simulink model "satellite_GVE_per_model_formation_sim"  (R2021a)
settings: Solver=VariableStepAuto  StartTime=0  StopTime=10800  FixedStep=1  RelTol=1e-3
values from neighbouring files (symbols this model uses):
  a_ini = (960e3+1019e3)/2+R_e    (= 7367700)    [Satellite_MPC3.m]
  Cd = 2.2    [Satellite_MPC3.m]
  e_ini = 0.0039866    [Satellite_MPC3.m]
  Form_dis = 1e3    (= 1000)    [Satellite_MPC3.m]
  i_ini = 82.9236/180*pi()    [Satellite_MPC3.m]
  J2 = 1082.63e-6    (= 0.00108263)    [Satellite_MPC3.m]
  K = 2    [Satellite_MPC3.m]
  kd = 0    [Satellite_MPC3.m]
  ki = 0    [Satellite_MPC3.m]
  kp = 4e-7    (= 4e-07)    [Satellite_MPC3.m]
  m_s = 27    [Satellite_MPC3.m]
  meu = G*m_e    (= 397865500000000)    [Satellite_MPC3.m]
  Ohm_ini = 272.9481/180*pi()    [Satellite_MPC3.m]
  p_solar = 4.65e-06    [Satellite_MPC3.m]
  R_e = 6378.2e3    (= 6378200)    [Satellite_MPC3.m]
  s = 0.2*0.2    (= 0.04)    [Satellite_MPC3.m]
  theta1_ini = 0    [Satellite_MPC3.m]
  theta2_ini = 1e-7    (= 1e-07)    [Satellite_MPC3.m]
  theta3_ini = 2e-7    (= 2e-07)    [Satellite_MPC3.m]
  theta_ini = 0    [Satellite_MPC3.m]
  u_lim = inf    [Satellite_MPC3.m]
  w_ini = 297.2910/180*pi()    [Satellite_MPC3.m]
libraries: pid_lib x3
(part 1 of 2)
settings Model: OrderedModelArguments=off  Creator=18214  LastModifiedBy=18214

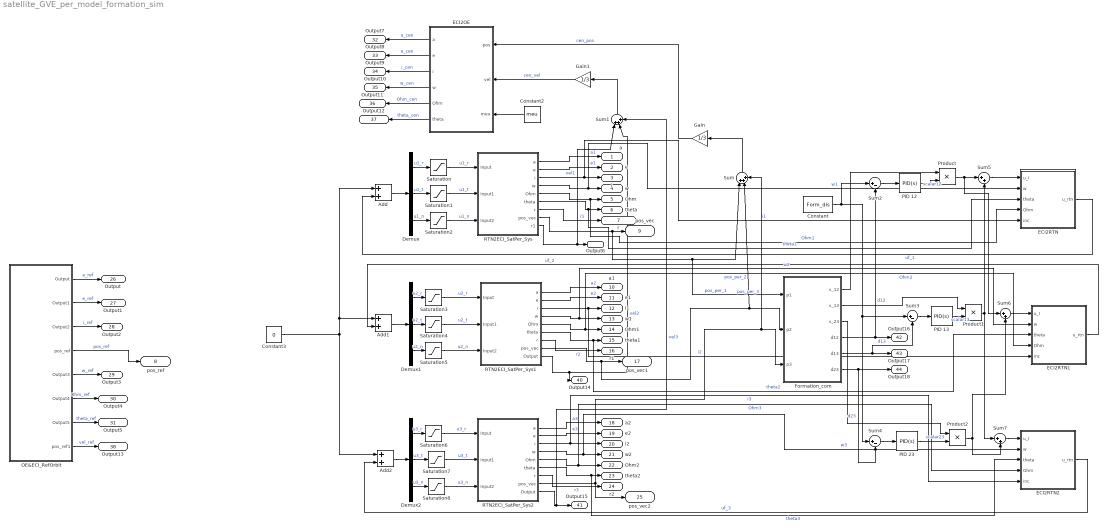
== system satellite_GVE_per_model_formation_sim ==
  Add : Sum
  Add1 : Sum
  Add2 : Sum
  Constant : Constant  Value=Form_dis
  Constant2 : Constant  Value=meu
  Constant3 : Constant  Value=0
  Demux : Demux  Outputs=3
  Demux1 : Demux  Outputs=3
  Demux2 : Demux  Outputs=3
  ECI2OE : MATLAB Function  TreatAsAtomicUnit=on
  ECI2RTN : MATLAB Function  TreatAsAtomicUnit=on
  ECI2RTN1 : MATLAB Function  TreatAsAtomicUnit=on
  ECI2RTN2 : MATLAB Function  TreatAsAtomicUnit=on
  Formation_com : MATLAB Function  TreatAsAtomicUnit=on
  Gain : Gain  Gain=1/3
  Gain1 : Gain  Gain=1/3
  OE&ECI_RefOrbit : Subsystem
  PID 12 : pid_lib/PID Controller  Controller=PID  Form=Parallel  TimeDomain=Continuous-time  UseExternalTs=off  SampleTime=-1  IntegratorMethod=Forward Euler  FilterMethod=Forward Euler  ControllerParametersSource=internal  P=kp  I=ki  D=kd  UseFilter=on  N=100  TunerSelectOption=Transfer Function Based (PID Tuner App)  InitialConditionSource=internal  InitialConditionForIntegrator=0  InitialConditionForFilter=0  DifferentiatorICPrevScaledInput=0  ExternalReset=none  TrackingMode=off  Kt=1  LimitOutput=off  SatLimitsSource=internal  UpperSaturationLimit=inf  LowerSaturationLimit=-inf  LinearizeAsGain=on  AntiWindupMode=none  Kb=1  POutMin=[]  POutMax=[]  IOutMin=[]  IOutMax=[]  DOutMin=[]  DOutMax=[]  NOutMin=[]  NOutMax=[]  SumOutMin=[]  SumOutMax=[]  SaturationOutMin=[]  SaturationOutMax=[]  PParamMin=[]  PParamMax=[]  IParamMin=[]  IParamMax=[]  DParamMin=[]  DParamMax=[]  NParamMin=[]  NParamMax=[]  KbParamMin=[]  KbParamMax=[]  KtParamMin=[]  KtParamMax=[]  KbOutMin=[]  KbOutMax=[]  KtOutMin=[]  KtOutMax=[]  IntegratorOutMin=[]  IntegratorOutMax=[]  FilterOutMin=[]  FilterOutMax=[]  SumI1OutMin=[]  SumI1OutMax=[]  SumI2OutMin=[]  SumI2OutMax=[]  SumI3OutMin=[]  SumI3OutMax=[]  SumI4OutMin=[]  SumI4OutMax=[]  SumDOutMin=[]  SumDOutMax=[]  DifferentiatorOutMin=[]  DifferentiatorOutMax=[]  FilterDiffOutCoefMin=[]  FilterDiffOutCoefMax=[]  ReciprocalOutMin=[]  ReciprocalOutMax=[]  SumDenOutMin=[]  SumDenOutMax=[]  SumNumOutMin=[]  SumNumOutMax=[]  DivideOutMin=[]  DivideOutMax=[]  UdiffTsProdOutMin=[]  UdiffTsProdOutMax=[]  NTsProdOutMin=[]  NTsProdOutMax=[]  UintegralTsProdOutMin=[]  UintegralTsProdOutMax=[]  UngainTsProdOutMin=[]  UngainTsProdOutMax=[]  IntegratorContinuousStateAttributes=''  IntegratorStateMustResolveToSignalObject=off  IntegratorRTWStateStorageClass=Auto  FilterContinuousStateAttributes=''  FilterStateMustResolveToSignalObject=off  FilterRTWStateStorageClass=Auto  ParallelPVariant=InternalParameters  IdealPVariant=Disabled  IVariant=InternalParameters  DVariant=InternalParameters  IntegratorVariant=Continuous  SatVariant=Disabled  AWVariant=Passthrough  PCopyVariant=Disabled  TRVariant=Disabled  FdbkBlocksVariant=Forward  IdealPFdbkVariant=Disabled  SatFdbkVariant=Disabled  DerivativeFilterVariant=ContFilter  NVariant=InternalParameters  NCopyVariant=Disabled  FilterICVariant=InternalICsFilter  IntegratorICVariant=InternalICs  ExternalResetVariant=Disabled  TRSumVariant=Passthrough  SumFdbkVariant=Disabled  SumVariant=Sum_PID  TsampFilterVariant=InternalTs  TsampNgainVariant=Passthrough  TsampIntegralVariant=Passthrough  ExternalSaturationOutDataTypeStr=Inherit: Same as second input
  PID 13 : pid_lib/PID Controller  Controller=PID  Form=Parallel  TimeDomain=Continuous-time  UseExternalTs=off  SampleTime=-1  IntegratorMethod=Forward Euler  FilterMethod=Forward Euler  ControllerParametersSource=internal  P=kp  I=ki  D=kd  UseFilter=on  N=100  TunerSelectOption=Transfer Function Based (PID Tuner App)  InitialConditionSource=internal  InitialConditionForIntegrator=0  InitialConditionForFilter=0  DifferentiatorICPrevScaledInput=0  ExternalReset=none  TrackingMode=off  Kt=1  LimitOutput=off  SatLimitsSource=internal  UpperSaturationLimit=inf  LowerSaturationLimit=-inf  LinearizeAsGain=on  AntiWindupMode=none  Kb=1  POutMin=[]  POutMax=[]  IOutMin=[]  IOutMax=[]  DOutMin=[]  DOutMax=[]  NOutMin=[]  NOutMax=[]  SumOutMin=[]  SumOutMax=[]  SaturationOutMin=[]  SaturationOutMax=[]  PParamMin=[]  PParamMax=[]  IParamMin=[]  IParamMax=[]  DParamMin=[]  DParamMax=[]  NParamMin=[]  NParamMax=[]  KbParamMin=[]  KbParamMax=[]  KtParamMin=[]  KtParamMax=[]  KbOutMin=[]  KbOutMax=[]  KtOutMin=[]  KtOutMax=[]  IntegratorOutMin=[]  IntegratorOutMax=[]  FilterOutMin=[]  FilterOutMax=[]  SumI1OutMin=[]  SumI1OutMax=[]  SumI2OutMin=[]  SumI2OutMax=[]  SumI3OutMin=[]  SumI3OutMax=[]  SumI4OutMin=[]  SumI4OutMax=[]  SumDOutMin=[]  SumDOutMax=[]  DifferentiatorOutMin=[]  DifferentiatorOutMax=[]  FilterDiffOutCoefMin=[]  FilterDiffOutCoefMax=[]  ReciprocalOutMin=[]  ReciprocalOutMax=[]  SumDenOutMin=[]  SumDenOutMax=[]  SumNumOutMin=[]  SumNumOutMax=[]  DivideOutMin=[]  DivideOutMax=[]  UdiffTsProdOutMin=[]  UdiffTsProdOutMax=[]  NTsProdOutMin=[]  NTsProdOutMax=[]  UintegralTsProdOutMin=[]  UintegralTsProdOutMax=[]  UngainTsProdOutMin=[]  UngainTsProdOutMax=[]  IntegratorContinuousStateAttributes=''  IntegratorStateMustResolveToSignalObject=off  IntegratorRTWStateStorageClass=Auto  FilterContinuousStateAttributes=''  FilterStateMustResolveToSignalObject=off  FilterRTWStateStorageClass=Auto  ParallelPVariant=InternalParameters  IdealPVariant=Disabled  IVariant=InternalParameters  DVariant=InternalParameters  IntegratorVariant=Continuous  SatVariant=Disabled  AWVariant=Passthrough  PCopyVariant=Disabled  TRVariant=Disabled  FdbkBlocksVariant=Forward  IdealPFdbkVariant=Disabled  SatFdbkVariant=Disabled  DerivativeFilterVariant=ContFilter  NVariant=InternalParameters  NCopyVariant=Disabled  FilterICVariant=InternalICsFilter  IntegratorICVariant=InternalICs  ExternalResetVariant=Disabled  TRSumVariant=Passthrough  SumFdbkVariant=Disabled  SumVariant=Sum_PID  TsampFilterVariant=InternalTs  TsampNgainVariant=Passthrough  TsampIntegralVariant=Passthrough  ExternalSaturationOutDataTypeStr=Inherit: Same as second input
  PID 23 : pid_lib/PID Controller  Controller=PID  Form=Parallel  TimeDomain=Continuous-time  UseExternalTs=off  SampleTime=-1  IntegratorMethod=Forward Euler  FilterMethod=Forward Euler  ControllerParametersSource=internal  P=kp  I=ki  D=kd  UseFilter=on  N=100  TunerSelectOption=Transfer Function Based (PID Tuner App)  InitialConditionSource=internal  InitialConditionForIntegrator=0  InitialConditionForFilter=0  DifferentiatorICPrevScaledInput=0  ExternalReset=none  TrackingMode=off  Kt=1  LimitOutput=off  SatLimitsSource=internal  UpperSaturationLimit=inf  LowerSaturationLimit=-inf  LinearizeAsGain=on  AntiWindupMode=none  Kb=1  POutMin=[]  POutMax=[]  IOutMin=[]  IOutMax=[]  DOutMin=[]  DOutMax=[]  NOutMin=[]  NOutMax=[]  SumOutMin=[]  SumOutMax=[]  SaturationOutMin=[]  SaturationOutMax=[]  PParamMin=[]  PParamMax=[]  IParamMin=[]  IParamMax=[]  DParamMin=[]  DParamMax=[]  NParamMin=[]  NParamMax=[]  KbParamMin=[]  KbParamMax=[]  KtParamMin=[]  KtParamMax=[]  KbOutMin=[]  KbOutMax=[]  KtOutMin=[]  KtOutMax=[]  IntegratorOutMin=[]  IntegratorOutMax=[]  FilterOutMin=[]  FilterOutMax=[]  SumI1OutMin=[]  SumI1OutMax=[]  SumI2OutMin=[]  SumI2OutMax=[]  SumI3OutMin=[]  SumI3OutMax=[]  SumI4OutMin=[]  SumI4OutMax=[]  SumDOutMin=[]  SumDOutMax=[]  DifferentiatorOutMin=[]  DifferentiatorOutMax=[]  FilterDiffOutCoefMin=[]  FilterDiffOutCoefMax=[]  ReciprocalOutMin=[]  ReciprocalOutMax=[]  SumDenOutMin=[]  SumDenOutMax=[]  SumNumOutMin=[]  SumNumOutMax=[]  DivideOutMin=[]  DivideOutMax=[]  UdiffTsProdOutMin=[]  UdiffTsProdOutMax=[]  NTsProdOutMin=[]  NTsProdOutMax=[]  UintegralTsProdOutMin=[]  UintegralTsProdOutMax=[]  UngainTsProdOutMin=[]  UngainTsProdOutMax=[]  IntegratorContinuousStateAttributes=''  IntegratorStateMustResolveToSignalObject=off  IntegratorRTWStateStorageClass=Auto  FilterContinuousStateAttributes=''  FilterStateMustResolveToSignalObject=off  FilterRTWStateStorageClass=Auto  ParallelPVariant=InternalParameters  IdealPVariant=Disabled  IVariant=InternalParameters  DVariant=InternalParameters  IntegratorVariant=Continuous  SatVariant=Disabled  AWVariant=Passthrough  PCopyVariant=Disabled  TRVariant=Disabled  FdbkBlocksVariant=Forward  IdealPFdbkVariant=Disabled  SatFdbkVariant=Disabled  DerivativeFilterVariant=ContFilter  NVariant=InternalParameters  NCopyVariant=Disabled  FilterICVariant=InternalICsFilter  IntegratorICVariant=InternalICs  ExternalResetVariant=Disabled  TRSumVariant=Passthrough  SumFdbkVariant=Disabled  SumVariant=Sum_PID  TsampFilterVariant=InternalTs  TsampNgainVariant=Passthrough  TsampIntegralVariant=Passthrough  ExternalSaturationOutDataTypeStr=Inherit: Same as second input
  Product : Product
  Product1 : Product
  Product2 : Product
  RTN2ECI_SatPer_Sys : Subsystem
  RTN2ECI_SatPer_Sys1 : Subsystem
  RTN2ECI_SatPer_Sys2 : Subsystem
  Saturation{,1..8} (9 alike) : Saturate  UpperLimit=u_lim  LowerLimit=-u_lim
  Sum : Sum  Inputs=|+++
  Sum1 : Sum  Inputs=|+++
  Sum2 : Sum  Inputs=|+-
  Sum3 : Sum  Inputs=|+-
  Sum4 : Sum  Inputs=|+-
  Sum5 : Sum  Inputs=|++
  Sum6 : Sum  Inputs=|++
  Sum7 : Sum  Inputs=|++
  a : Outport
  e : Outport  Port=2
  i : Outport  Port=3
  w : Outport  Port=4
  Ohm : Outport  Port=5
  theta : Outport  Port=6
  r : Outport  Port=7
  pos_ref : Outport  Port=8
  pos_vec : Outport  Port=9
  a1 : Outport  Port=10
  e1 : Outport  Port=11
  i1 : Outport  Port=12
  w1 : Outport  Port=13
  Ohm1 : Outport  Port=14
  theta1 : Outport  Port=15
  r1 : Outport  Port=16
  pos_vec1 : Outport  Port=17
  a2 : Outport  Port=18
  e2 : Outport  Port=19
  i2 : Outport  Port=20
  w2 : Outport  Port=21
  Ohm2 : Outport  Port=22
  theta2 : Outport  Port=23
  r2 : Outport  Port=24
  pos_vec2 : Outport  Port=25
  Output : Outport  Port=26
  Output1 : Outport  Port=27
  Output2 : Outport  Port=28
  Output3 : Outport  Port=29
  Output4 : Outport  Port=30
  Output5 : Outport  Port=31
  Output7 : Outport  Port=32
  Output8 : Outport  Port=33
  Output9 : Outport  Port=34
  Output10 : Outport  Port=35
  Output11 : Outport  Port=36
  Output12 : Outport  Port=37
  Output13 : Outport  Port=38
  Output6 : Outport  Port=39
  Output14 : Outport  Port=40
  Output15 : Outport  Port=41
  Output16 : Outport  Port=42
  Output17 : Outport  Port=43
  Output18 : Outport  Port=44
  wires:
  Saturation/1 -> RTN2ECI_SatPer_Sys/1(Input)  "u1_r"
  Saturation1/1 -> RTN2ECI_SatPer_Sys/2(Input1)  "u1_t"
  Saturation2/1 -> RTN2ECI_SatPer_Sys/3(Input2)  "u1_n"
  RTN2ECI_SatPer_Sys/1(a) -> a/1  "a1"
  RTN2ECI_SatPer_Sys/2(e) -> e/1  "e1"
  RTN2ECI_SatPer_Sys/3(i) -> ECI2RTN/5(inc), i/1  "i1"
  RTN2ECI_SatPer_Sys/4(w) -> ECI2RTN/2(w), w/1  "w1"
  RTN2ECI_SatPer_Sys/5(Ohm) -> ECI2RTN/4(Ohm), Ohm/1  "Ohm1"
  RTN2ECI_SatPer_Sys/6(theta) -> ECI2RTN/3(theta), theta/1  "theta1"
  RTN2ECI_SatPer_Sys/7(r) -> r/1  "r1"
  RTN2ECI_SatPer_Sys/8(pos_vec) -> Formation_com/1(p1), Sum/1, pos_vec/1  "pos_per_1"
  RTN2ECI_SatPer_Sys1/8(pos_vec) -> Formation_com/2(p2), Sum/2, pos_vec1/1  "pos_per_2"
  RTN2ECI_SatPer_Sys1/7(r) -> r1/1  "r2"
  RTN2ECI_SatPer_Sys1/6(theta) -> ECI2RTN1/3(theta), theta1/1  "theta2"
  RTN2ECI_SatPer_Sys1/5(Ohm) -> ECI2RTN1/4(Ohm), Ohm1/1  "Ohm2"
  RTN2ECI_SatPer_Sys1/4(w) -> ECI2RTN1/2(w), w1/1  "w2"
  RTN2ECI_SatPer_Sys1/3(i) -> ECI2RTN1/5(inc), i1/1  "i2"
  RTN2ECI_SatPer_Sys1/2(e) -> e1/1  "e2"
  RTN2ECI_SatPer_Sys1/1(a) -> a1/1  "a2"
  Saturation5/1 -> RTN2ECI_SatPer_Sys1/3(Input2)  "u2_n"
  Saturation4/1 -> RTN2ECI_SatPer_Sys1/2(Input1)  "u2_t"
  Saturation3/1 -> RTN2ECI_SatPer_Sys1/1(Input)  "u2_r"
  Saturation6/1 -> RTN2ECI_SatPer_Sys2/1(Input)  "u3_r"
  Saturation7/1 -> RTN2ECI_SatPer_Sys2/2(Input1)  "u3_t"
  Saturation8/1 -> RTN2ECI_SatPer_Sys2/3(Input2)  "u3_n"
  RTN2ECI_SatPer_Sys2/1(a) -> a2/1  "a3"
  RTN2ECI_SatPer_Sys2/2(e) -> e2/1  "e3"
  RTN2ECI_SatPer_Sys2/3(i) -> ECI2RTN2/5(inc), i2/1  "i3"
  RTN2ECI_SatPer_Sys2/4(w) -> ECI2RTN2/2(w), w2/1  "w3"
  RTN2ECI_SatPer_Sys2/5(Ohm) -> ECI2RTN2/4(Ohm), Ohm2/1  "Ohm3"
  RTN2ECI_SatPer_Sys2/6(theta) -> ECI2RTN2/3(theta), theta2/1  "theta3"
  RTN2ECI_SatPer_Sys2/7(r) -> r2/1  "r3"
  RTN2ECI_SatPer_Sys2/8(pos_vec) -> pos_vec2/1, Formation_com/3(p3), Sum/3  "pos_per_3"
  OE&ECI_RefOrbit/1(Output) -> Output/1  "a_ref"
  OE&ECI_RefOrbit/2(Output1) -> Output1/1  "e_ref"
  OE&ECI_RefOrbit/3(Output2) -> Output2/1  "i_ref"
  OE&ECI_RefOrbit/4(pos_ref) -> pos_ref/1  "pos_ref"
  OE&ECI_RefOrbit/5(Output3) -> Output3/1  "w_ref"
  OE&ECI_RefOrbit/6(Output4) -> Output4/1  "Ohm_ref"
  OE&ECI_RefOrbit/7(Output5) -> Output5/1  "theta_ref"
  Constant/1 -> Sum3/1, Sum4/1, Sum2/1
  Sum/1 -> Gain/1
  Add/1 -> Demux/1
  Add1/1 -> Demux1/1
  Add2/1 -> Demux2/1
  Constant3/1 -> Add2/1, Add/1, Add1/1
  Gain/1 -> ECI2OE/1(pos)  "cen_pos"
  Constant2/1 -> ECI2OE/3(meu)
  ECI2OE/1(a) -> Output7/1  "a_cen"
  ECI2OE/2(e) -> Output8/1  "e_cen"
  ECI2OE/3(i) -> Output9/1  "i_cen"
  ECI2OE/4(w) -> Output10/1  "w_cen"
  ECI2OE/5(Ohm) -> Output11/1  "Ohm_cen"
  ECI2OE/6(theta) -> Output12/1  "theta_cen"
  OE&ECI_RefOrbit/8(pos_ref1) -> Output13/1  "vel_ref"
  RTN2ECI_SatPer_Sys/9(r1) -> Sum1/1, Output6/1  "vel1"
  RTN2ECI_SatPer_Sys1/9(Output) -> Sum1/2, Output14/1  "vel2"
  RTN2ECI_SatPer_Sys2/9(Output) -> Sum1/3, Output15/1  "vel3"
  Gain1/1 -> ECI2OE/2(vel)  "cen_vel"
  Sum1/1 -> Gain1/1
  ECI2RTN/1(u_rtn) -> Add/2  "uf_1"
  Sum3/1 -> PID 13/1
  ECI2RTN1/1(u_rtn) -> Add1/2  "uf_2"
  Demux/1 -> Saturation/1  "u1_r"
  Demux/2 -> Saturation1/1  "u1_t"
  Demux/3 -> Saturation2/1  "u1_n"
  Demux1/1 -> Saturation3/1  "u2_r"
  Demux1/2 -> Saturation4/1  "u2_t"
  Demux1/3 -> Saturation5/1  "u2_n"
  Demux2/1 -> Saturation6/1  "u3_r"
  Demux2/2 -> Saturation7/1  "u3_t"
  Demux2/3 -> Saturation8/1  "u3_n"
  Sum4/1 -> PID 23/1
  ECI2RTN2/1(u_rtn) -> Add2/2  "uf_3"
  Formation_com/4(d12) -> Output16/1, Sum2/2  "d12"
  Formation_com/5(d13) -> Sum3/2, Output17/1  "d13"
  Formation_com/6(d23) -> Sum4/2, Output18/1  "d23"
  Sum5/1 -> ECI2RTN/1(u_I)
  Product1/1 -> Sum5/2, Sum7/1
  Sum7/1 -> ECI2RTN2/1(u_I)
  Sum2/1 -> PID 12/1
  PID 12/1 -> Product/2  "scalar12"
  Formation_com/1(v_12) -> Product/1
  PID 13/1 -> Product1/2  "scalar13"
  Formation_com/2(v_13) -> Product1/1
  PID 23/1 -> Product2/2  "scalar23"
  Formation_com/3(v_23) -> Product2/1
  Product/1 -> Sum6/1, Sum5/1
  Sum6/1 -> ECI2RTN1/1(u_I)
  Product2/1 -> Sum6/2, Sum7/2

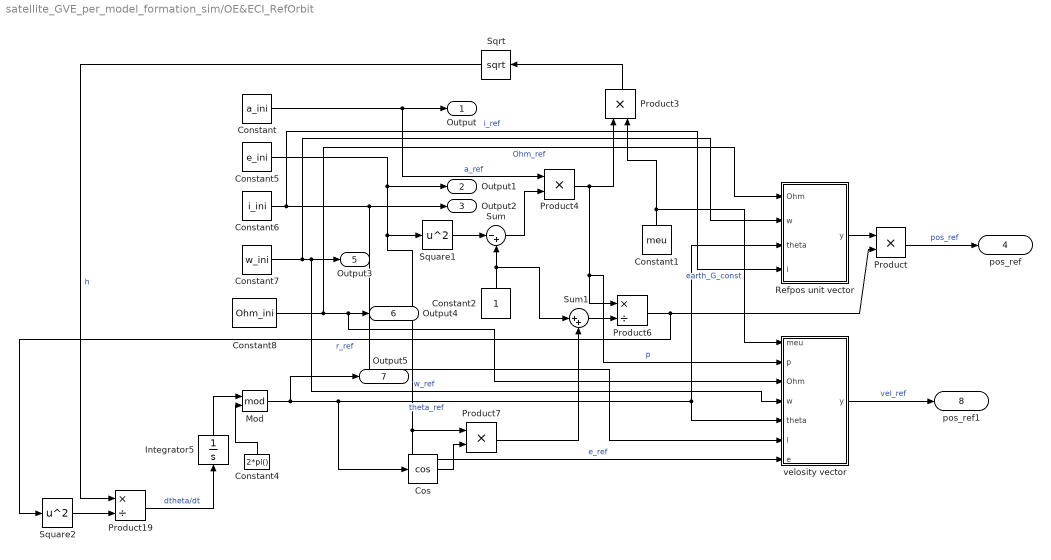
== system satellite_GVE_per_model_formation_sim/OE&ECI_RefOrbit ==
  Constant : Constant  Value=a_ini
  Constant1 : Constant  Value=meu
  Constant2 : Constant
  Constant4 : Constant  Value=2*pi()
  Constant5 : Constant  Value=e_ini
  Constant6 : Constant  Value=i_ini
  Constant7 : Constant  Value=w_ini
  Constant8 : Constant  Value=Ohm_ini
  Cos : Trigonometry  Operator=cos
  Integrator5 : Integrator  InitialCondition=theta_ini
  Mod : Math  Operator=mod  SaturateOnIntegerOverflow=on
  Product{,3..4,7} (4 alike) : Product
  Product19 : Product  Inputs=*/
  Product6 : Product  Inputs=*/
  Refpos unit vector : MATLAB Function  TreatAsAtomicUnit=on
  Sqrt : Sqrt  SaturateOnIntegerOverflow=on
  Square1 : Math  Operator=square  SaturateOnIntegerOverflow=on
  Square2 : Math  Operator=square  SaturateOnIntegerOverflow=on
  Sum : Sum  Inputs=|-+
  Sum1 : Sum  Inputs=|++
  velosity vector : MATLAB Function  TreatAsAtomicUnit=on
  Output : Outport
  Output1 : Outport  Port=2
  Output2 : Outport  Port=3
  pos_ref : Outport  Port=4
  Output3 : Outport  Port=5
  Output4 : Outport  Port=6
  Output5 : Outport  Port=7
  pos_ref1 : Outport  Port=8
  wires:
  Constant/1 -> Output/1, Product4/1  "a_ref"
  Constant6/1 -> velosity vector/6(i), Output2/1, Refpos unit vector/4(i)  "i_ref"
  Constant7/1 -> velosity vector/4(w), Output3/1, Refpos unit vector/2(w)  "w_ref"
  Product6/1 -> Product/2, Square2/1  "r_ref"
  Constant8/1 -> velosity vector/3(Ohm), Output4/1, Refpos unit vector/1(Ohm)  "Ohm_ref"
  Constant2/1 -> Sum/2, Sum1/1
  Refpos unit vector/1(y) -> Product/1
  Product/1 -> pos_ref/1  "pos_ref"
  Product7/1 -> Sum1/2
  Product4/1 -> velosity vector/2(p), Product6/1, Product3/1  "p"
  Cos/1 -> Product7/2
  Mod/1 -> Output5/1, velosity vector/5(theta), Refpos unit vector/3(theta), Cos/1  "theta_ref"
  Integrator5/1 -> Mod/1
  Square1/1 -> Sum/1
  Sqrt/1 -> Product19/1  "h"
  Constant5/1 -> Output1/1, Product7/1, velosity vector/7(e), Square1/1  "e_ref"
  Sum/1 -> Product4/2
  Constant4/1 -> Mod/2
  Product3/1 -> Sqrt/1
  Product19/1 -> Integrator5/1  "dtheta/dt"
  Constant1/1 -> Product3/2, velosity vector/1(meu)  "earth_G_const"
  Square2/1 -> Product19/2
  Sum1/1 -> Product6/2
  velosity vector/1(y) -> pos_ref1/1  "vel_ref"

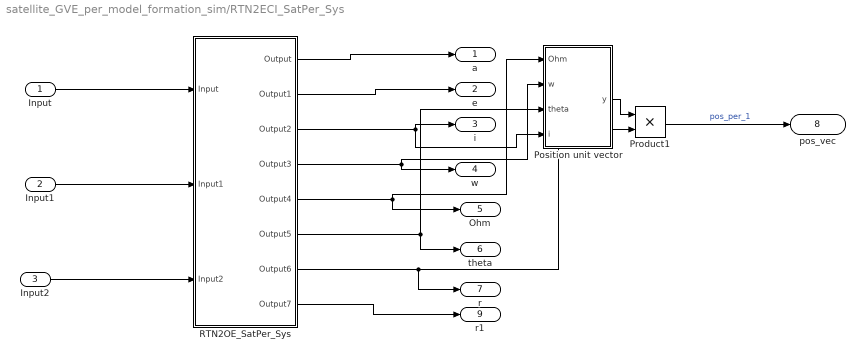
== system satellite_GVE_per_model_formation_sim/RTN2ECI_SatPer_Sys ==
  Input : Inport
  Input1 : Inport  Port=2
  Input2 : Inport  Port=3
  Position unit vector : MATLAB Function  TreatAsAtomicUnit=on
  Product1 : Product
  RTN2OE_SatPer_Sys : Subsystem
  a : Outport
  e : Outport  Port=2
  i : Outport  Port=3
  w : Outport  Port=4
  Ohm : Outport  Port=5
  theta : Outport  Port=6
  r : Outport  Port=7
  pos_vec : Outport  Port=8
  r1 : Outport  Port=9
  wires:
  Position unit vector/1(y) -> Product1/1
  RTN2OE_SatPer_Sys/6(Output5) -> theta/1, Position unit vector/3(theta)
  RTN2OE_SatPer_Sys/4(Output3) -> w/1, Position unit vector/2(w)
  Product1/1 -> pos_vec/1  "pos_per_1"
  RTN2OE_SatPer_Sys/2(Output1) -> e/1
  RTN2OE_SatPer_Sys/5(Output4) -> Ohm/1, Position unit vector/1(Ohm)
  RTN2OE_SatPer_Sys/7(Output6) -> r/1, Product1/2
  RTN2OE_SatPer_Sys/1(Output) -> a/1
  RTN2OE_SatPer_Sys/3(Output2) -> Position unit vector/4(i), i/1
  Input/1 -> RTN2OE_SatPer_Sys/1(Input)
  Input1/1 -> RTN2OE_SatPer_Sys/2(Input1)
  Input2/1 -> RTN2OE_SatPer_Sys/3(Input2)
  RTN2OE_SatPer_Sys/8(Output7) -> r1/1

== system satellite_GVE_per_model_formation_sim/RTN2ECI_SatPer_Sys1 ==
  Input : Inport
  Input1 : Inport  Port=2
  Input2 : Inport  Port=3
  Position unit vector : MATLAB Function  TreatAsAtomicUnit=on
  Product1 : Product
  RTN2OE_SatPer_Sys : Subsystem
  a : Outport
  e : Outport  Port=2
  i : Outport  Port=3
  w : Outport  Port=4
  Ohm : Outport  Port=5
  theta : Outport  Port=6
  r : Outport  Port=7
  pos_vec : Outport  Port=8
  Output : Outport  Port=9
  wires:
  RTN2OE_SatPer_Sys/3(Output2) -> Position unit vector/4(i), i/1
  RTN2OE_SatPer_Sys/1(Output) -> a/1
  RTN2OE_SatPer_Sys/7(Output6) -> r/1, Product1/2
  RTN2OE_SatPer_Sys/5(Output4) -> Position unit vector/1(Ohm), Ohm/1
  RTN2OE_SatPer_Sys/2(Output1) -> e/1
  Product1/1 -> pos_vec/1  "pos_per_2"
  RTN2OE_SatPer_Sys/4(Output3) -> Position unit vector/2(w), w/1
  RTN2OE_SatPer_Sys/6(Output5) -> theta/1, Position unit vector/3(theta)
  Position unit vector/1(y) -> Product1/1
  Input/1 -> RTN2OE_SatPer_Sys/1(Input)
  Input1/1 -> RTN2OE_SatPer_Sys/2(Input1)
  Input2/1 -> RTN2OE_SatPer_Sys/3(Input2)
  RTN2OE_SatPer_Sys/8(Output7) -> Output/1

== system satellite_GVE_per_model_formation_sim/RTN2ECI_SatPer_Sys2 ==
  Input : Inport
  Input1 : Inport  Port=2
  Input2 : Inport  Port=3
  Position unit vector : MATLAB Function  TreatAsAtomicUnit=on
  Product1 : Product
  RTN2OE_SatPer_Sys : Subsystem
  a : Outport
  e : Outport  Port=2
  i : Outport  Port=3
  w : Outport  Port=4
  Ohm : Outport  Port=5
  theta : Outport  Port=6
  r : Outport  Port=7
  pos_vec : Outport  Port=8
  Output : Outport  Port=9
  wires:
  Position unit vector/1(y) -> Product1/1
  RTN2OE_SatPer_Sys/6(Output5) -> theta/1, Position unit vector/3(theta)
  RTN2OE_SatPer_Sys/4(Output3) -> w/1, Position unit vector/2(w)
  Product1/1 -> pos_vec/1  "pos_per_3"
  RTN2OE_SatPer_Sys/2(Output1) -> e/1
  RTN2OE_SatPer_Sys/5(Output4) -> Ohm/1, Position unit vector/1(Ohm)
  RTN2OE_SatPer_Sys/7(Output6) -> r/1, Product1/2
  RTN2OE_SatPer_Sys/1(Output) -> a/1
  RTN2OE_SatPer_Sys/3(Output2) -> i/1, Position unit vector/4(i)
  Input/1 -> RTN2OE_SatPer_Sys/1(Input)
  Input1/1 -> RTN2OE_SatPer_Sys/2(Input1)
  Input2/1 -> RTN2OE_SatPer_Sys/3(Input2)
  RTN2OE_SatPer_Sys/8(Output7) -> Output/1

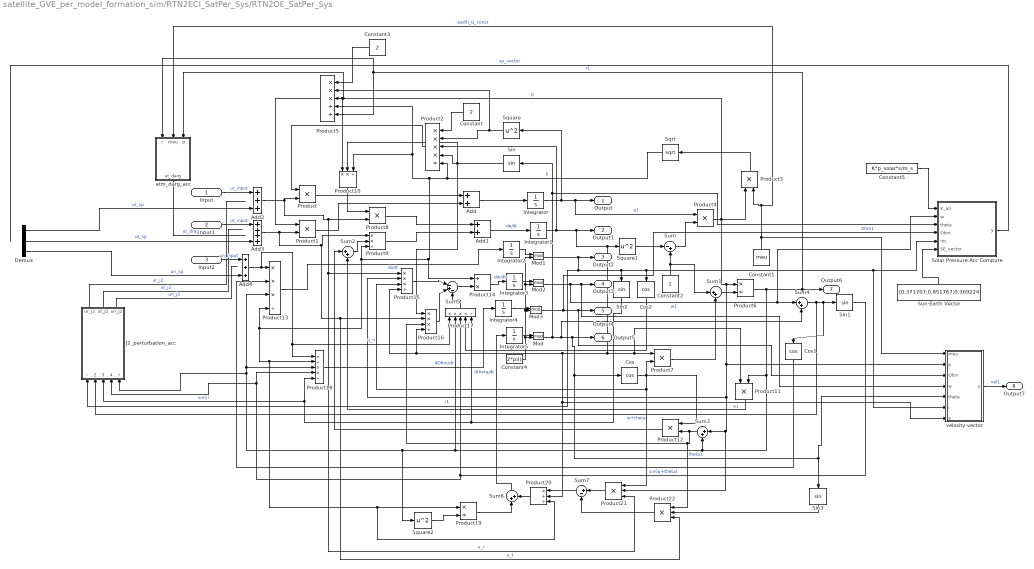
== system satellite_GVE_per_model_formation_sim/RTN2ECI_SatPer_Sys/RTN2OE_SatPer_Sys ==
  Input : Inport
  Input1 : Inport  Port=2
  Input2 : Inport  Port=3
  Add : Sum
  Add1 : Sum
  Add2 : Sum  Inputs=+++
  Add3 : Sum  Inputs=++++
  Add4 : Sum  Inputs=+++
  Constant : Constant  Value=2
  Constant1 : Constant  Value=meu
  Constant2 : Constant
  Constant3 : Constant  Value=2
  Constant4 : Constant  Value=2*pi()
  Constant5 : Constant  Value=K*p_solar*s/m_s
  Cos : Trigonometry  Operator=cos
  Cos1 : Trigonometry  Operator=cos
  Cos2 : Trigonometry  Operator=cos
  Demux : Demux  Outputs=3
  Integrator : Integrator  InitialCondition=a_ini  LimitOutput=on  LowerSaturationLimit=R_e
  Integrator1 : Integrator  InitialCondition=e_ini  LimitOutput=on  UpperSaturationLimit=1  LowerSaturationLimit=0
  Integrator2 : Integrator  InitialCondition=i_ini  UpperSaturationLimit=312.5963  LowerSaturationLimit=-312.5963
  Integrator3 : Integrator  InitialCondition=w_ini  UpperSaturationLimit=312.5963  LowerSaturationLimit=-312.5963
  Integrator4 : Integrator  InitialCondition=Ohm_ini  UpperSaturationLimit=312.5963  LowerSaturationLimit=-312.5963
  Integrator5 : Integrator  InitialCondition=theta1_ini  UpperSaturationLimit=312.5963  LowerSaturationLimit=-312.5963
  J2_perturbation_acc : Subsystem
  Mod{,1..3} (4 alike) : Math  Operator=mod  SaturateOnIntegerOverflow=on
  Product{,1,3..4,7..8,11..12} (8 alike) : Product
  Product10 : Product  Inputs=**/
  Product13 : Product  Inputs=***/
  Product14 : Product  Inputs=/*
  Product15 : Product  Inputs=***/
  Product16 : Product  Inputs=***/
  Product17 : Product  Inputs=****/
  Product18 : Product  Inputs=*/**/
  Product19 : Product  Inputs=*/
  Product2 : Product  Inputs=****/
  Product20 : Product  Inputs=*//
  Product21 : Product  Inputs=***
  Product22 : Product  Inputs=***
  Product5 : Product  Inputs=***//
  Product6 : Product  Inputs=*/
  Product9 : Product  Inputs=**/
  Sin{,1..3} (4 alike) : Trigonometry
  Solar Pressure Acc Compute : MATLAB Function  TreatAsAtomicUnit=on
  Sqrt : Sqrt  SaturateOnIntegerOverflow=on
  Square : Math  Operator=square  SaturateOnIntegerOverflow=on
  Square1 : Math  Operator=square  SaturateOnIntegerOverflow=on
  Square2 : Math  Operator=square  SaturateOnIntegerOverflow=on
  Sum : Sum  Inputs=|-+
  Sum{1..4,6} (5 alike) : Sum  Inputs=|++
  Sum5 : Sum  Inputs=|-+-
  Sum7 : Sum  Inputs=|+-
  Sun-Earth Vector : Constant  Value=[0.371707;0.851767;0.369224]
  atm_darg_acc : Subsystem
  velosity vector : MATLAB Function  TreatAsAtomicUnit=on
  Output : Outport
  Output1 : Outport  Port=2
  Output2 : Outport  Port=3
  Output3 : Outport  Port=4
  Output4 : Outport  Port=5
  Output5 : Outport  Port=6
  Output6 : Outport  Port=7
  Output7 : Outport  Port=8
  wires:
  Integrator/1 -> Output/1, Product4/1, Square/1  "a1"
  Square2/1 -> Product19/2
  Product2/1 -> Product/1
  Mod/1 -> Sin/1, Solar Pressure Acc Compute/3(theta), Output5/1, Sin3/1, velosity vector/5(theta), Cos/1, Sum4/2  "theta1"
  Sin1/1 -> Product18/4, J2_perturbation_acc/4(sin(w+theta)), Product17/3  "sin(w+theta)"
  Product21/1 -> Sum7/1
  Sum5/1 -> Product14/2
  Cos/1 -> Product21/1, Product15/3, Product12/1, Product7/2
  Product4/1 -> Product15/2, Product21/2, Sum3/1, velosity vector/2(p), Product6/1, atm_darg_acc/3(p), Product10/1, Product5/3, Product3/1  "p"
  Cos2/1 -> Product17/4
  Sin/1 -> Product16/1, Product10/2, Product2/4
  Sqrt/1 -> Product10/3, Product5/4, Product14/1, Product13/4, Product20/3, Product19/1, Product18/2, Product9/3, Product2/5  "h"
  Product12/1 -> Sum2/1
  Sum/1 -> Product4/2
  Sum3/1 -> Product22/1, Product16/3, Product12/2
  Sum7/1 -> Product20/1
  Product1/1 -> Add/2
  Product22/1 -> Sum7/2
  Add2/1 -> Product/2, Product21/3, Product15/1, Product8/2  "u_r"
  Product7/1 -> Sum1/2
  Product5/1 -> Product1/1
  Sin3/1 -> Product22/2
  Product15/1 -> Sum5/1
  Integrator1/1 -> Product2/3, Output1/1, Square1/1, Product7/1, Product11/1, Product20/2, velosity vector/7(e), Product16/4, Product15/4  "e1"
  Sum1/1 -> Product6/2
  Cos1/1 -> Product13/2
  Product19/1 -> Sum6/1
  Product8/1 -> Add1/1
  Product6/1 -> atm_darg_acc/1(r), Product5/5, Output6/1, Square2/1, J2_perturbation_acc/5(r), Product13/3, Product18/3, Product17/2, Sum3/2, Product11/2  "r1"
  Constant2/1 -> Sum/2, Sum1/1
  Square/1 -> Product5/2, Product2/2
  Product11/1 -> Sum2/2
  Product/1 -> Add/1
  Mod1/1 -> Output2/1, velosity vector/6(i), Solar Pressure Acc Compute/5(inc), Cos2/1, Sin2/1, J2_perturbation_acc/1(i)  "i1"
  Sin2/1 -> Product18/5, J2_perturbation_acc/3(sin(i)), Product17/5  "sin(i)"
  Product17/1 -> Sum5/3
  Product16/1 -> Sum5/2
  Sum6/1 -> Integrator5/1  "dtheta/dt"
  Product10/1 -> Product8/1
  Product9/1 -> Add1/2
  Sum4/1 -> Sin1/1, Cos1/1, J2_perturbation_acc/2(w+theta)  "w+theta"
  Product20/1 -> Sum6/2
  Mod2/1 -> Solar Pressure Acc Compute/2(w), Sum4/1, velosity vector/4(w), Output3/1  "w1"
  Add3/1 -> Product22/3, Product16/2, Product9/1, Product1/2  "u_t"
  Constant/1 -> Product2/1
  Sum2/1 -> Product9/2
  Product14/1 -> Integrator3/1  "dw/dt"
  Square1/1 -> Sum/1
  Add4/1 -> Product18/1, Product17/1, Product13/1  "u_n"
  Product13/1 -> Integrator2/1  "di/dt"
  Constant1/1 -> velosity vector/1(meu), Product3/2, atm_darg_acc/2(meu)  "earth_G_const"
  Mod3/1 -> Solar Pressure Acc Compute/4(Ohm), velosity vector/3(Ohm), Output4/1  "Ohm1"
  Product18/1 -> Integrator4/1  "dOhm/dt"
  Add1/1 -> Integrator1/1  "de/dt"
  Constant3/1 -> Product5/1
  Product3/1 -> Sqrt/1
  Integrator5/1 -> Mod/1
  Constant4/1 -> Mod3/2, Mod2/2, Mod1/2, Mod/2
  Input/1 -> Add2/1  "ur_input"
  Input1/1 -> Add3/1  "ut_input"
  Input2/1 -> Add4/1  "un_input"
  atm_darg_acc/1(ut_darg) -> ?  "ut_drag"
  J2_perturbation_acc/1(ur_J2) -> ?  "ur_j2"
  J2_perturbation_acc/2(ut_J2) -> ?  "ut_j2"
  J2_perturbation_acc/3(un_J2) -> ?  "un_j2"
  Add/1 -> Integrator/1
  Integrator2/1 -> Mod1/1
  Integrator3/1 -> Mod2/1
  Integrator4/1 -> Mod3/1
  Sun-Earth Vector/1 -> Solar Pressure Acc Compute/6(SE_vector)
  Constant5/1 -> Solar Pressure Acc Compute/1(K_all)
  Solar Pressure Acc Compute/1(y) -> ?  "sp_vector"
  Demux/1 -> Add2/3  "ur_sp"
  Demux/2 -> Add3/4  "ut_sp"
  Demux/3 -> Add4/3  "un_sp"
  velosity vector/1(y) -> Output7/1  "vel1"

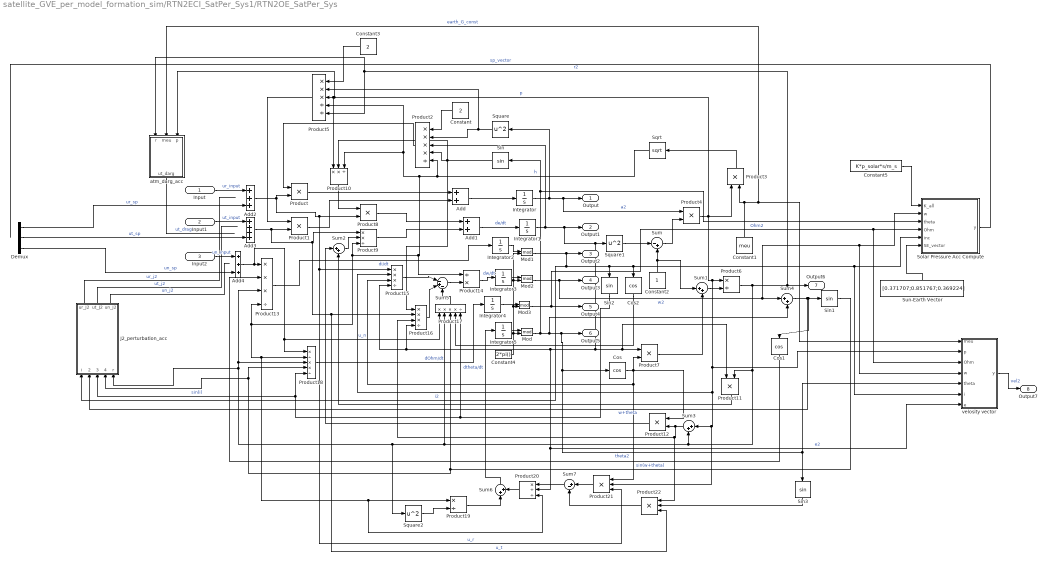
== system satellite_GVE_per_model_formation_sim/RTN2ECI_SatPer_Sys1/RTN2OE_SatPer_Sys ==
  Input : Inport
  Input1 : Inport  Port=2
  Input2 : Inport  Port=3
  Add : Sum
  Add1 : Sum
  Add2 : Sum  Inputs=+++
  Add3 : Sum  Inputs=++++
  Add4 : Sum  Inputs=+++
  Constant : Constant  Value=2
  Constant1 : Constant  Value=meu
  Constant2 : Constant
  Constant3 : Constant  Value=2
  Constant4 : Constant  Value=2*pi()
  Constant5 : Constant  Value=K*p_solar*s/m_s
  Cos : Trigonometry  Operator=cos
  Cos1 : Trigonometry  Operator=cos
  Cos2 : Trigonometry  Operator=cos
  Demux : Demux  Outputs=3
  Integrator : Integrator  InitialCondition=a_ini  LimitOutput=on  LowerSaturationLimit=R_e
  Integrator1 : Integrator  InitialCondition=e_ini  LimitOutput=on  UpperSaturationLimit=1  LowerSaturationLimit=0
  Integrator2 : Integrator  InitialCondition=i_ini  UpperSaturationLimit=312.5963  LowerSaturationLimit=-312.5963
  Integrator3 : Integrator  InitialCondition=w_ini  UpperSaturationLimit=312.5963  LowerSaturationLimit=-312.5963
  Integrator4 : Integrator  InitialCondition=Ohm_ini  UpperSaturationLimit=312.5963  LowerSaturationLimit=-312.5963
  Integrator5 : Integrator  InitialCondition=theta2_ini  UpperSaturationLimit=312.5963  LowerSaturationLimit=-312.5963
  J2_perturbation_acc : Subsystem
  Mod{,1..3} (4 alike) : Math  Operator=mod  SaturateOnIntegerOverflow=on
  Product{,1,3..4,7..8,11..12} (8 alike) : Product
  Product10 : Product  Inputs=**/
  Product13 : Product  Inputs=***/
  Product14 : Product  Inputs=/*
  Product15 : Product  Inputs=***/
  Product16 : Product  Inputs=***/
  Product17 : Product  Inputs=****/
  Product18 : Product  Inputs=*/**/
  Product19 : Product  Inputs=*/
  Product2 : Product  Inputs=****/
  Product20 : Product  Inputs=*//
  Product21 : Product  Inputs=***
  Product22 : Product  Inputs=***
  Product5 : Product  Inputs=***//
  Product6 : Product  Inputs=*/
  Product9 : Product  Inputs=**/
  Sin{,1..3} (4 alike) : Trigonometry
  Solar Pressure Acc Compute : MATLAB Function  TreatAsAtomicUnit=on
  Sqrt : Sqrt  SaturateOnIntegerOverflow=on
  Square : Math  Operator=square  SaturateOnIntegerOverflow=on
  Square1 : Math  Operator=square  SaturateOnIntegerOverflow=on
  Square2 : Math  Operator=square  SaturateOnIntegerOverflow=on
  Sum : Sum  Inputs=|-+
  Sum{1..4,6} (5 alike) : Sum  Inputs=|++
  Sum5 : Sum  Inputs=|-+-
  Sum7 : Sum  Inputs=|+-
  Sun-Earth Vector : Constant  Value=[0.371707;0.851767;0.369224]
  atm_darg_acc : Subsystem
  velosity vector : MATLAB Function  TreatAsAtomicUnit=on
  Output : Outport
  Output1 : Outport  Port=2
  Output2 : Outport  Port=3
  Output3 : Outport  Port=4
  Output4 : Outport  Port=5
  Output5 : Outport  Port=6
  Output6 : Outport  Port=7
  Output7 : Outport  Port=8
  wires:
  Demux/3 -> Add4/3  "un_sp"
  Demux/2 -> Add3/4  "ut_sp"
  Demux/1 -> Add2/3  "ur_sp"
  Solar Pressure Acc Compute/1(y) -> ?  "sp_vector"
  Constant5/1 -> Solar Pressure Acc Compute/1(K_all)
  Sun-Earth Vector/1 -> Solar Pressure Acc Compute/6(SE_vector)
  Integrator4/1 -> Mod3/1
  Integrator3/1 -> Mod2/1
  Integrator2/1 -> Mod1/1
  Add/1 -> Integrator/1
  J2_perturbation_acc/3(un_J2) -> ?  "un_j2"
  J2_perturbation_acc/2(ut_J2) -> ?  "ut_j2"
  J2_perturbation_acc/1(ur_J2) -> ?  "ur_j2"
  atm_darg_acc/1(ut_darg) -> ?  "ut_drag"
  Input2/1 -> Add4/1  "un_input"
  Input1/1 -> Add3/1  "ut_input"
  Input/1 -> Add2/1  "ur_input"
  Constant4/1 -> Mod/2, Mod1/2, Mod2/2, Mod3/2
  Integrator5/1 -> Mod/1
  Product3/1 -> Sqrt/1
  Constant3/1 -> Product5/1
  Add1/1 -> Integrator1/1  "de/dt"
  Product18/1 -> Integrator4/1  "dOhm/dt"
  Mod3/1 -> Output4/1, velosity vector/3(Ohm), Solar Pressure Acc Compute/4(Ohm)  "Ohm2"
  Constant1/1 -> Product3/2, velosity vector/1(meu), atm_darg_acc/2(meu)  "earth_G_const"
  Product13/1 -> Integrator2/1  "di/dt"
  Add4/1 -> Product13/1, Product17/1, Product18/1  "u_n"
  Square1/1 -> Sum/1
  Product14/1 -> Integrator3/1  "dw/dt"
  Sum2/1 -> Product9/2
  Constant/1 -> Product2/1
  Add3/1 -> Product1/2, Product9/1, Product16/2, Product22/3  "u_t"
  Mod2/1 -> Output3/1, Sum4/1, velosity vector/4(w), Solar Pressure Acc Compute/2(w)  "w2"
  Product20/1 -> Sum6/2
  Sum4/1 -> J2_perturbation_acc/2(w+theta), Cos1/1, Sin1/1  "w+theta"
  Product9/1 -> Add1/2
  Product10/1 -> Product8/1
  Sum6/1 -> Integrator5/1  "dtheta/dt"
  Product16/1 -> Sum5/2
  Product17/1 -> Sum5/3
  Sin2/1 -> Product17/5, J2_perturbation_acc/3(sin(i)), Product18/5  "sin(i)"
  Mod1/1 -> J2_perturbation_acc/1(i), Sin2/1, Cos2/1, Solar Pressure Acc Compute/5(inc), velosity vector/6(i), Output2/1  "i2"
  Product/1 -> Add/1
  Product11/1 -> Sum2/2
  Square/1 -> Product2/2, Product5/2
  Constant2/1 -> Sum1/1, Sum/2
  Product6/1 -> Product11/2, Sum3/2, Product17/2, Product18/3, Product13/3, J2_perturbation_acc/5(r), Square2/1, Output6/1, Product5/5, atm_darg_acc/1(r)  "r2"
  Product8/1 -> Add1/1
  Product19/1 -> Sum6/1
  Cos1/1 -> Product13/2
  Sum1/1 -> Product6/2
  Integrator1/1 -> Product15/4, Product16/4, Product20/2, velosity vector/7(e), Product11/1, Product7/1, Square1/1, Output1/1, Product2/3  "e2"
  Product15/1 -> Sum5/1
  Sin3/1 -> Product22/2
  Product5/1 -> Product1/1
  Product7/1 -> Sum1/2
  Add2/1 -> Product8/2, Product15/1, Product21/3, Product/2  "u_r"
  Product22/1 -> Sum7/2
  Product1/1 -> Add/2
  Sum7/1 -> Product20/1
  Sum3/1 -> Product12/2, Product16/3, Product22/1
  Sum/1 -> Product4/2
  Product12/1 -> Sum2/1
  Sqrt/1 -> Product2/5, Product9/3, Product18/2, Product19/1, Product20/3, Product13/4, Product14/1, Product5/4, Product10/3  "h"
  Sin/1 -> Product2/4, Product10/2, Product16/1
  Cos2/1 -> Product17/4
  Product4/1 -> Product3/1, Product5/3, Product10/1, atm_darg_acc/3(p), Product6/1, velosity vector/2(p), Sum3/1, Product21/2, Product15/2  "p"
  Cos/1 -> Product7/2, Product12/1, Product15/3, Product21/1
  Sum5/1 -> Product14/2
  Product21/1 -> Sum7/1
  Sin1/1 -> Product17/3, J2_perturbation_acc/4(sin(w+theta)), Product18/4  "sin(w+theta)"
  Mod/1 -> Sum4/2, Cos/1, velosity vector/5(theta), Sin3/1, Output5/1, Solar Pressure Acc Compute/3(theta), Sin/1  "theta2"
  Product2/1 -> Product/1
  Square2/1 -> Product19/2
  Integrator/1 -> Square/1, Product4/1, Output/1  "a2"
  velosity vector/1(y) -> Output7/1  "vel2"

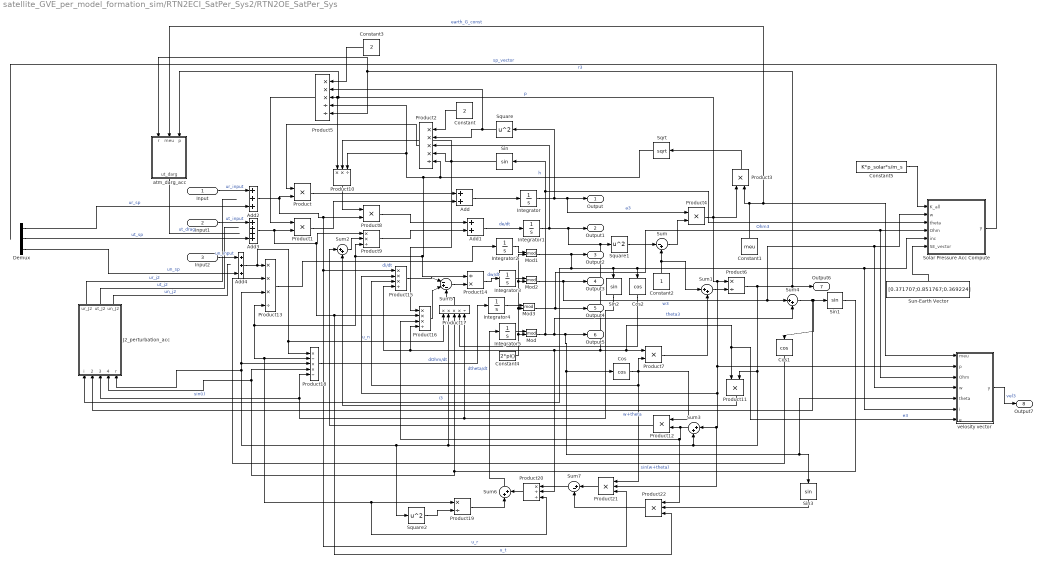
== system satellite_GVE_per_model_formation_sim/RTN2ECI_SatPer_Sys2/RTN2OE_SatPer_Sys ==
  Input : Inport
  Input1 : Inport  Port=2
  Input2 : Inport  Port=3
  Add : Sum
  Add1 : Sum
  Add2 : Sum  Inputs=+++
  Add3 : Sum  Inputs=++++
  Add4 : Sum  Inputs=+++
  Constant : Constant  Value=2
  Constant1 : Constant  Value=meu
  Constant2 : Constant
  Constant3 : Constant  Value=2
  Constant4 : Constant  Value=2*pi()
  Constant5 : Constant  Value=K*p_solar*s/m_s
  Cos : Trigonometry  Operator=cos
  Cos1 : Trigonometry  Operator=cos
  Cos2 : Trigonometry  Operator=cos
  Demux : Demux  Outputs=3
  Integrator : Integrator  InitialCondition=a_ini  LimitOutput=on  LowerSaturationLimit=R_e
  Integrator1 : Integrator  InitialCondition=e_ini  LimitOutput=on  UpperSaturationLimit=1  LowerSaturationLimit=0
  Integrator2 : Integrator  InitialCondition=i_ini  UpperSaturationLimit=312.5963  LowerSaturationLimit=-312.5963
  Integrator3 : Integrator  InitialCondition=w_ini  UpperSaturationLimit=312.5963  LowerSaturationLimit=-312.5963
  Integrator4 : Integrator  InitialCondition=Ohm_ini  UpperSaturationLimit=312.5963  LowerSaturationLimit=-312.5963
  Integrator5 : Integrator  InitialCondition=theta3_ini  UpperSaturationLimit=312.5963  LowerSaturationLimit=-312.5963
  J2_perturbation_acc : Subsystem
  Mod{,1..3} (4 alike) : Math  Operator=mod  SaturateOnIntegerOverflow=on
  Product{,1,3..4,7..8,11..12} (8 alike) : Product
  Product10 : Product  Inputs=**/
  Product13 : Product  Inputs=***/
  Product14 : Product  Inputs=/*
  Product15 : Product  Inputs=***/
  Product16 : Product  Inputs=***/
  Product17 : Product  Inputs=****/
  Product18 : Product  Inputs=*/**/
  Product19 : Product  Inputs=*/
  Product2 : Product  Inputs=****/
  Product20 : Product  Inputs=*//
  Product21 : Product  Inputs=***
  Product22 : Product  Inputs=***
  Product5 : Product  Inputs=***//
  Product6 : Product  Inputs=*/
  Product9 : Product  Inputs=**/
  Sin{,1..3} (4 alike) : Trigonometry
  Solar Pressure Acc Compute : MATLAB Function  TreatAsAtomicUnit=on
  Sqrt : Sqrt  SaturateOnIntegerOverflow=on
  Square : Math  Operator=square  SaturateOnIntegerOverflow=on
  Square1 : Math  Operator=square  SaturateOnIntegerOverflow=on
  Square2 : Math  Operator=square  SaturateOnIntegerOverflow=on
  Sum : Sum  Inputs=|-+
  Sum{1..4,6} (5 alike) : Sum  Inputs=|++
  Sum5 : Sum  Inputs=|-+-
  Sum7 : Sum  Inputs=|+-
  Sun-Earth Vector : Constant  Value=[0.371707;0.851767;0.369224]
  atm_darg_acc : Subsystem
  velosity vector : MATLAB Function  TreatAsAtomicUnit=on
  Output : Outport
  Output1 : Outport  Port=2
  Output2 : Outport  Port=3
  Output3 : Outport  Port=4
  Output4 : Outport  Port=5
  Output5 : Outport  Port=6
  Output6 : Outport  Port=7
  Output7 : Outport  Port=8
  wires:
  Integrator/1 -> Output/1, Product4/1, Square/1  "a3"
  Square2/1 -> Product19/2
  Product2/1 -> Product/1
  Mod/1 -> Sin/1, Solar Pressure Acc Compute/3(theta), Output5/1, velosity vector/5(theta), Sin3/1, Cos/1, Sum4/2  "theta3"
  Sin1/1 -> Product18/4, J2_perturbation_acc/4(sin(w+theta)), Product17/3  "sin(w+theta)"
  Product21/1 -> Sum7/1
  Sum5/1 -> Product14/2
  Cos/1 -> Product21/1, Product15/3, Product12/1, Product7/2
  Product4/1 -> velosity vector/2(p), Product15/2, Product21/2, Sum3/1, Product6/1, atm_darg_acc/3(p), Product10/1, Product5/3, Product3/1  "p"
  Cos2/1 -> Product17/4
  Sin/1 -> Product16/1, Product10/2, Product2/4
  Sqrt/1 -> Product10/3, Product5/4, Product14/1, Product13/4, Product20/3, Product19/1, Product18/2, Product9/3, Product2/5  "h"
  Product12/1 -> Sum2/1
  Sum/1 -> Product4/2
  Sum3/1 -> Product22/1, Product16/3, Product12/2
  Sum7/1 -> Product20/1
  Product1/1 -> Add/2
  Product22/1 -> Sum7/2
  Add2/1 -> Product/2, Product21/3, Product15/1, Product8/2  "u_r"
  Product7/1 -> Sum1/2
  Product5/1 -> Product1/1
  Sin3/1 -> Product22/2
  Product15/1 -> Sum5/1
  Integrator1/1 -> Product2/3, Output1/1, Square1/1, Product7/1, velosity vector/7(e), Product11/1, Product20/2, Product16/4, Product15/4  "e3"
  Sum1/1 -> Product6/2
  Cos1/1 -> Product13/2
  Product19/1 -> Sum6/1
  Product8/1 -> Add1/1
  Product6/1 -> atm_darg_acc/1(r), Product5/5, Output6/1, Square2/1, J2_perturbation_acc/5(r), Product13/3, Product18/3, Product17/2, Sum3/2, Product11/2  "r3"
  Constant2/1 -> Sum/2, Sum1/1
  Square/1 -> Product5/2, Product2/2
  Product11/1 -> Sum2/2
  Product/1 -> Add/1
  Mod1/1 -> Output2/1, velosity vector/6(i), Solar Pressure Acc Compute/5(inc), Cos2/1, Sin2/1, J2_perturbation_acc/1(i)  "i3"
  Sin2/1 -> Product18/5, J2_perturbation_acc/3(sin(i)), Product17/5  "sin(i)"
  Product17/1 -> Sum5/3
  Product16/1 -> Sum5/2
  Sum6/1 -> Integrator5/1  "dtheta/dt"
  Product10/1 -> Product8/1
  Product9/1 -> Add1/2
  Sum4/1 -> Sin1/1, Cos1/1, J2_perturbation_acc/2(w+theta)  "w+theta"
  Product20/1 -> Sum6/2
  Mod2/1 -> velosity vector/4(w), Solar Pressure Acc Compute/2(w), Sum4/1, Output3/1  "w3"
  Add3/1 -> Product22/3, Product16/2, Product9/1, Product1/2  "u_t"
  Constant/1 -> Product2/1
  Sum2/1 -> Product9/2
  Product14/1 -> Integrator3/1  "dw/dt"
  Square1/1 -> Sum/1
  Add4/1 -> Product18/1, Product17/1, Product13/1  "u_n"
  Product13/1 -> Integrator2/1  "di/dt"
  Constant1/1 -> velosity vector/1(meu), atm_darg_acc/2(meu), Product3/2  "earth_G_const"
  Mod3/1 -> velosity vector/3(Ohm), Solar Pressure Acc Compute/4(Ohm), Output4/1  "Ohm3"
  Product18/1 -> Integrator4/1  "dOhm/dt"
  Add1/1 -> Integrator1/1  "de/dt"
  Constant3/1 -> Product5/1
  Product3/1 -> Sqrt/1
  Integrator5/1 -> Mod/1
  Constant4/1 -> Mod3/2, Mod2/2, Mod1/2, Mod/2
  Input/1 -> Add2/1  "ur_input"
  Input1/1 -> Add3/1  "ut_input"
  Input2/1 -> Add4/1  "un_input"
  atm_darg_acc/1(ut_darg) -> ?  "ut_drag"
  J2_perturbation_acc/1(ur_J2) -> ?  "ur_j2"
  J2_perturbation_acc/2(ut_J2) -> ?  "ut_j2"
  J2_perturbation_acc/3(un_J2) -> ?  "un_j2"
  Add/1 -> Integrator/1
  Integrator2/1 -> Mod1/1
  Integrator3/1 -> Mod2/1
  Integrator4/1 -> Mod3/1
  Sun-Earth Vector/1 -> Solar Pressure Acc Compute/6(SE_vector)
  Constant5/1 -> Solar Pressure Acc Compute/1(K_all)
  Solar Pressure Acc Compute/1(y) -> ?  "sp_vector"
  Demux/1 -> Add2/3  "ur_sp"
  Demux/2 -> Add3/4  "ut_sp"
  Demux/3 -> Add4/3  "un_sp"
  velosity vector/1(y) -> Output7/1  "vel3"

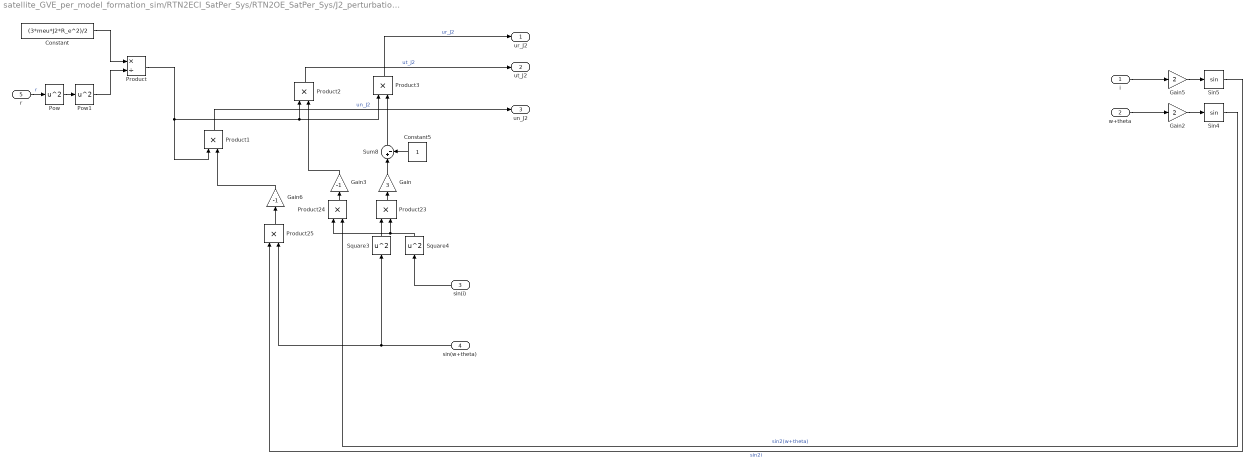
== system satellite_GVE_per_model_formation_sim/RTN2ECI_SatPer_Sys/RTN2OE_SatPer_Sys/J2_perturbation_acc ==
  i : Inport
  w+theta : Inport  Port=2
  sin(i) : Inport  Port=3
  sin(w+theta) : Inport  Port=4
  r : Inport  Port=5
  Constant : Constant  Value=(3*meu*J2*R_e^2)/2
  Constant5 : Constant
  Gain : Gain  Gain=3
  Gain2 : Gain  Gain=2
  Gain3 : Gain  Gain=-1
  Gain5 : Gain  Gain=2
  Gain6 : Gain  Gain=-1
  Pow : Math  Operator=square  RndMeth=Zero  SaturateOnIntegerOverflow=on
  Pow1 : Math  Operator=square  RndMeth=Zero  SaturateOnIntegerOverflow=on
  Product : Product  Inputs=*/
  Product{1..3,23..25} (6 alike) : Product
  Sin4 : Trigonometry
  Sin5 : Trigonometry
  Square3 : Math  Operator=square  SaturateOnIntegerOverflow=on
  Square4 : Math  Operator=square  SaturateOnIntegerOverflow=on
  Sum8 : Sum  Inputs=|+-
  ur_J2 : Outport
  ut_J2 : Outport  Port=2
  un_J2 : Outport  Port=3
  wires:
  Gain6/1 -> Product1/2
  Square4/1 -> Product23/2, Product24/1
  i/1 -> Gain5/1
  Square3/1 -> Product23/1
  Sin4/1 -> Product24/2  "sin2(w+theta)"
  Sum8/1 -> Product3/2
  Product3/1 -> ur_J2/1  "ur_J2"
  Gain5/1 -> Sin5/1
  Gain3/1 -> Product2/2
  w+theta/1 -> Gain2/1
  Gain/1 -> Sum8/1
  Product23/1 -> Gain/1
  sin(w+theta)/1 -> Product25/2, Square3/1
  Constant5/1 -> Sum8/2
  Sin5/1 -> Product25/1  "sin2i"
  Gain2/1 -> Sin4/1
  Product25/1 -> Gain6/1
  Product24/1 -> Gain3/1
  Product2/1 -> ut_J2/1  "ut_J2"
  sin(i)/1 -> Square4/1
  Product1/1 -> un_J2/1  "un_J2"
  r/1 -> Pow/1  "r"
  Pow1/1 -> Product/2
  Constant/1 -> Product/1
  Product/1 -> Product3/1, Product2/1, Product1/1
  Pow/1 -> Pow1/1

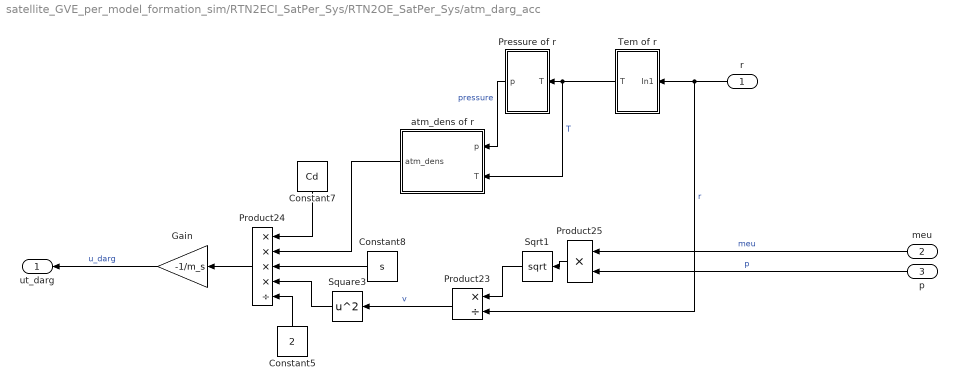
== system satellite_GVE_per_model_formation_sim/RTN2ECI_SatPer_Sys/RTN2OE_SatPer_Sys/atm_darg_acc ==
  r : Inport
  meu : Inport  Port=2
  p : Inport  Port=3
  Constant5 : Constant  Value=2
  Constant7 : Constant  Value=Cd
  Constant8 : Constant  Value=s
  Gain : Gain  Gain=-1/m_s
  Pressure of r : Subsystem
  Product23 : Product  Inputs=*/
  Product24 : Product  Inputs=****/
  Product25 : Product
  Sqrt1 : Sqrt  SaturateOnIntegerOverflow=on
  Square3 : Math  Operator=square  SaturateOnIntegerOverflow=on
  Tem of r : Subsystem
  atm_dens of r : Subsystem
  ut_darg : Outport
  wires:
  Tem of r/1(T) -> atm_dens of r/2(T), Pressure of r/1(T)  "T"
  Product24/1 -> Gain/1
  r/1 -> Product23/2, Tem of r/1(In1)  "r"
  Product25/1 -> Sqrt1/1
  Square3/1 -> Product24/4
  meu/1 -> Product25/1  "meu"
  Product23/1 -> Square3/1  "v"
  Constant7/1 -> Product24/1
  Sqrt1/1 -> Product23/1
  Pressure of r/1(p) -> atm_dens of r/1(p)  "pressure"
  Constant5/1 -> Product24/5
  atm_dens of r/1(atm_dens) -> Product24/2
  Constant8/1 -> Product24/3
  Gain/1 -> ut_darg/1  "u_darg"
  p/1 -> Product25/2  "p"

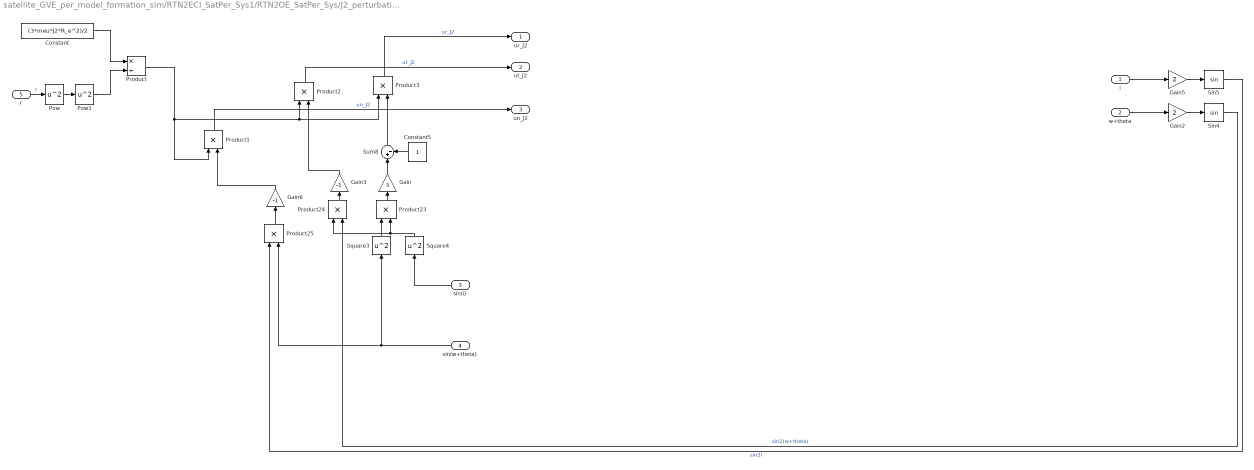
== system satellite_GVE_per_model_formation_sim/RTN2ECI_SatPer_Sys1/RTN2OE_SatPer_Sys/J2_perturbation_acc ==
  i : Inport
  w+theta : Inport  Port=2
  sin(i) : Inport  Port=3
  sin(w+theta) : Inport  Port=4
  r : Inport  Port=5
  Constant : Constant  Value=(3*meu*J2*R_e^2)/2
  Constant5 : Constant
  Gain : Gain  Gain=3
  Gain2 : Gain  Gain=2
  Gain3 : Gain  Gain=-1
  Gain5 : Gain  Gain=2
  Gain6 : Gain  Gain=-1
  Pow : Math  Operator=square  RndMeth=Zero  SaturateOnIntegerOverflow=on
  Pow1 : Math  Operator=square  RndMeth=Zero  SaturateOnIntegerOverflow=on
  Product : Product  Inputs=*/
  Product{1..3,23..25} (6 alike) : Product
  Sin4 : Trigonometry
  Sin5 : Trigonometry
  Square3 : Math  Operator=square  SaturateOnIntegerOverflow=on
  Square4 : Math  Operator=square  SaturateOnIntegerOverflow=on
  Sum8 : Sum  Inputs=|+-
  ur_J2 : Outport
  ut_J2 : Outport  Port=2
  un_J2 : Outport  Port=3
  wires:
  Pow/1 -> Pow1/1
  Product/1 -> Product1/1, Product2/1, Product3/1
  Constant/1 -> Product/1
  Pow1/1 -> Product/2
  r/1 -> Pow/1  "r"
  Product1/1 -> un_J2/1  "un_J2"
  sin(i)/1 -> Square4/1
  Product2/1 -> ut_J2/1  "ut_J2"
  Product24/1 -> Gain3/1
  Product25/1 -> Gain6/1
  Gain2/1 -> Sin4/1
  Sin5/1 -> Product25/1  "sin2i"
  Constant5/1 -> Sum8/2
  sin(w+theta)/1 -> Square3/1, Product25/2
  Product23/1 -> Gain/1
  Gain/1 -> Sum8/1
  w+theta/1 -> Gain2/1
  Gain3/1 -> Product2/2
  Gain5/1 -> Sin5/1
  Product3/1 -> ur_J2/1  "ur_J2"
  Sum8/1 -> Product3/2
  Sin4/1 -> Product24/2  "sin2(w+theta)"
  Square3/1 -> Product23/1
  i/1 -> Gain5/1
  Square4/1 -> Product24/1, Product23/2
  Gain6/1 -> Product1/2

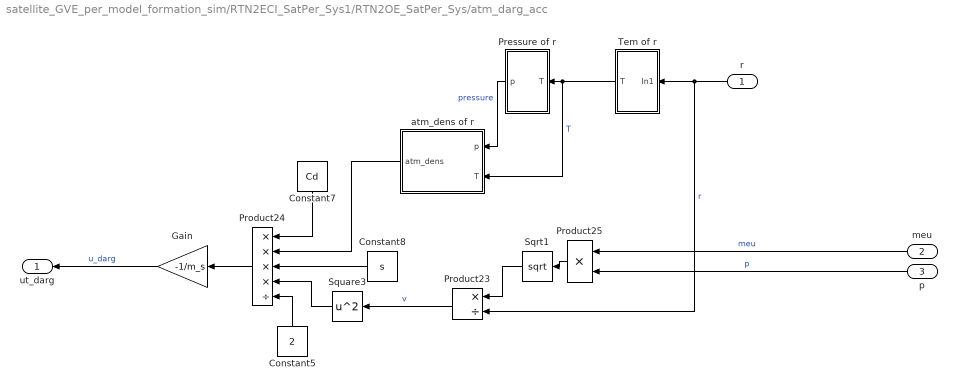
== system satellite_GVE_per_model_formation_sim/RTN2ECI_SatPer_Sys1/RTN2OE_SatPer_Sys/atm_darg_acc ==
  r : Inport
  meu : Inport  Port=2
  p : Inport  Port=3
  Constant5 : Constant  Value=2
  Constant7 : Constant  Value=Cd
  Constant8 : Constant  Value=s
  Gain : Gain  Gain=-1/m_s
  Pressure of r : Subsystem
  Product23 : Product  Inputs=*/
  Product24 : Product  Inputs=****/
  Product25 : Product
  Sqrt1 : Sqrt  SaturateOnIntegerOverflow=on
  Square3 : Math  Operator=square  SaturateOnIntegerOverflow=on
  Tem of r : Subsystem
  atm_dens of r : Subsystem
  ut_darg : Outport
  wires:
  p/1 -> Product25/2  "p"
  Gain/1 -> ut_darg/1  "u_darg"
  Constant8/1 -> Product24/3
  atm_dens of r/1(atm_dens) -> Product24/2
  Constant5/1 -> Product24/5
  Pressure of r/1(p) -> atm_dens of r/1(p)  "pressure"
  Sqrt1/1 -> Product23/1
  Constant7/1 -> Product24/1
  Product23/1 -> Square3/1  "v"
  meu/1 -> Product25/1  "meu"
  Square3/1 -> Product24/4
  Product25/1 -> Sqrt1/1
  r/1 -> Tem of r/1(In1), Product23/2  "r"
  Product24/1 -> Gain/1
  Tem of r/1(T) -> Pressure of r/1(T), atm_dens of r/2(T)  "T"

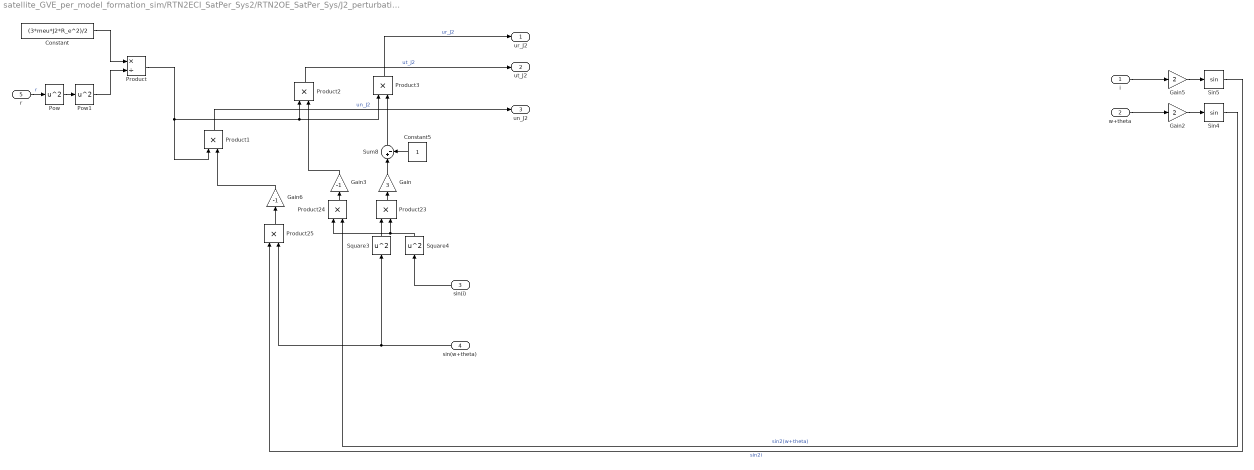
== system satellite_GVE_per_model_formation_sim/RTN2ECI_SatPer_Sys2/RTN2OE_SatPer_Sys/J2_perturbation_acc ==
  i : Inport
  w+theta : Inport  Port=2
  sin(i) : Inport  Port=3
  sin(w+theta) : Inport  Port=4
  r : Inport  Port=5
  Constant : Constant  Value=(3*meu*J2*R_e^2)/2
  Constant5 : Constant
  Gain : Gain  Gain=3
  Gain2 : Gain  Gain=2
  Gain3 : Gain  Gain=-1
  Gain5 : Gain  Gain=2
  Gain6 : Gain  Gain=-1
  Pow : Math  Operator=square  RndMeth=Zero  SaturateOnIntegerOverflow=on
  Pow1 : Math  Operator=square  RndMeth=Zero  SaturateOnIntegerOverflow=on
  Product : Product  Inputs=*/
  Product{1..3,23..25} (6 alike) : Product
  Sin4 : Trigonometry
  Sin5 : Trigonometry
  Square3 : Math  Operator=square  SaturateOnIntegerOverflow=on
  Square4 : Math  Operator=square  SaturateOnIntegerOverflow=on
  Sum8 : Sum  Inputs=|+-
  ur_J2 : Outport
  ut_J2 : Outport  Port=2
  un_J2 : Outport  Port=3
  wires:
  Gain6/1 -> Product1/2
  Square4/1 -> Product23/2, Product24/1
  i/1 -> Gain5/1
  Square3/1 -> Product23/1
  Sin4/1 -> Product24/2  "sin2(w+theta)"
  Sum8/1 -> Product3/2
  Product3/1 -> ur_J2/1  "ur_J2"
  Gain5/1 -> Sin5/1
  Gain3/1 -> Product2/2
  w+theta/1 -> Gain2/1
  Gain/1 -> Sum8/1
  Product23/1 -> Gain/1
  sin(w+theta)/1 -> Product25/2, Square3/1
  Constant5/1 -> Sum8/2
  Sin5/1 -> Product25/1  "sin2i"
  Gain2/1 -> Sin4/1
  Product25/1 -> Gain6/1
  Product24/1 -> Gain3/1
  Product2/1 -> ut_J2/1  "ut_J2"
  sin(i)/1 -> Square4/1
  Product1/1 -> un_J2/1  "un_J2"
  r/1 -> Pow/1  "r"
  Pow1/1 -> Product/2
  Constant/1 -> Product/1
  Product/1 -> Product3/1, Product2/1, Product1/1
  Pow/1 -> Pow1/1

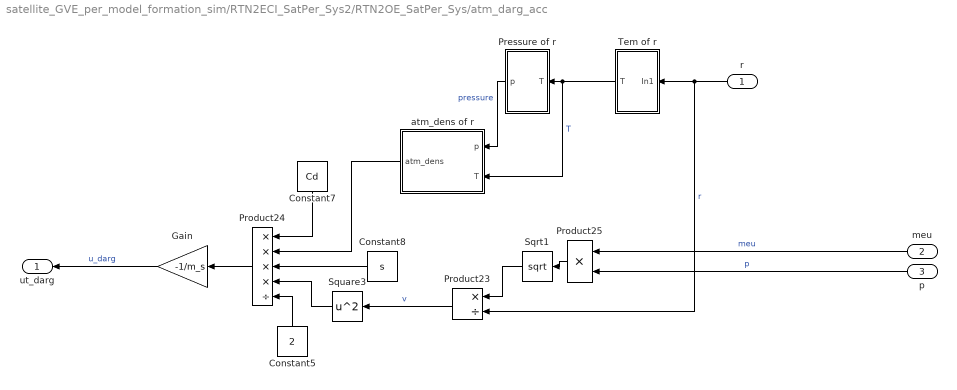
== system satellite_GVE_per_model_formation_sim/RTN2ECI_SatPer_Sys2/RTN2OE_SatPer_Sys/atm_darg_acc ==
  r : Inport
  meu : Inport  Port=2
  p : Inport  Port=3
  Constant5 : Constant  Value=2
  Constant7 : Constant  Value=Cd
  Constant8 : Constant  Value=s
  Gain : Gain  Gain=-1/m_s
  Pressure of r : Subsystem
  Product23 : Product  Inputs=*/
  Product24 : Product  Inputs=****/
  Product25 : Product
  Sqrt1 : Sqrt  SaturateOnIntegerOverflow=on
  Square3 : Math  Operator=square  SaturateOnIntegerOverflow=on
  Tem of r : Subsystem
  atm_dens of r : Subsystem
  ut_darg : Outport
  wires:
  Tem of r/1(T) -> atm_dens of r/2(T), Pressure of r/1(T)  "T"
  Product24/1 -> Gain/1
  r/1 -> Product23/2, Tem of r/1(In1)  "r"
  Product25/1 -> Sqrt1/1
  Square3/1 -> Product24/4
  meu/1 -> Product25/1  "meu"
  Product23/1 -> Square3/1  "v"
  Constant7/1 -> Product24/1
  Sqrt1/1 -> Product23/1
  Pressure of r/1(p) -> atm_dens of r/1(p)  "pressure"
  Constant5/1 -> Product24/5
  atm_dens of r/1(atm_dens) -> Product24/2
  Constant8/1 -> Product24/3
  Gain/1 -> ut_darg/1  "u_darg"
  p/1 -> Product25/2  "p"

== system satellite_GVE_per_model_formation_sim/RTN2ECI_SatPer_Sys/RTN2OE_SatPer_Sys/atm_darg_acc/Pressure of r ==
  T : Inport
  Constant : Constant  Value=2.448
  Constant5 : Constant  Value=273.1
  Constant7 : Constant  Value=216.6
  Constant8 : Constant  Value=11.388
  Math Function : Math  Operator=pow  SaturateOnIntegerOverflow=on
  Product : Product  Inputs=*/
  Product23 : Product  Inputs=*/
  Sum8 : Sum  Inputs=|++
  p : Outport
  wires:
  Constant5/1 -> Sum8/2
  Product/1 -> p/1  "p"
  T/1 -> Sum8/1
  Constant8/1 -> Math Function/1
  Sum8/1 -> Product23/1
  Constant7/1 -> Product23/2
  Product23/1 -> Math Function/2
  Math Function/1 -> Product/2
  Constant/1 -> Product/1

== system satellite_GVE_per_model_formation_sim/RTN2ECI_SatPer_Sys/RTN2OE_SatPer_Sys/atm_darg_acc/Tem of r ==
  In1 : Inport
  Constant5 : Constant  Value=-131.21
  Gain : Gain  Gain=0.00299
  Sum8 : Sum  Inputs=|++
  T : Outport
  wires:
  Sum8/1 -> T/1  "T"
  Gain/1 -> Sum8/1
  Constant5/1 -> Sum8/2
  In1/1 -> Gain/1

== system satellite_GVE_per_model_formation_sim/RTN2ECI_SatPer_Sys/RTN2OE_SatPer_Sys/atm_darg_acc/atm_dens of r ==
  p : Inport
  T : Inport  Port=2
  Constant5 : Constant  Value=0.2869
  Constant7 : Constant  Value=273.1
  Product23 : Product  Inputs=*//
  Sum8 : Sum  Inputs=|++
  atm_dens : Outport
  wires:
  T/1 -> Sum8/1
  Constant5/1 -> Product23/3
  Sum8/1 -> Product23/2
  Constant7/1 -> Sum8/2
  Product23/1 -> atm_dens/1  "atm_dens"
  p/1 -> Product23/1
